simulink model "uz_ParameterID"  (R2021a)
settings: Solver=FixedStepDiscrete  StartTime=0.0  StopTime=160  FixedStep=0.000005  RelTol=1e-3  EnableMultiTasking=on
model workspace (MATLAB code in the model file):
  | cmdLim = Simulink.Parameter;
  | cmdLim.Value = 15;
  | cmdLim.Description = 'Limit for controlling the maximum surface command angle.';
  | cmdLim.Min = 0;
  | cmdLim.Max = 90;
  | cmdLim.DocUnits = 'deg';
  | 
  | dispGain = Simulink.Parameter;
  | dispGain.Value = 0.75;
  | dispGain.Description = 'Gain applied to the displacement error.';
  | dispGain.Min = 0;
  | dispGain.Max = [];
  | dispGain.DocUnits = 'deg/sec/deg';
  | 
  | dispLim = Simulink.Parameter;
  | dispLim.Value = 30;
  | dispLim.Description = 'Limit for controlling the maximum commanded angle.';
  | dispLim.Min = 0;
  | dispLim.Max = 180;
  | dispLim.DocUnits = 'deg';
  | 
  | intGain = Simulink.Parameter;
  | intGain.Value = 0.5;
  | intGain.Description = 'Gain applied to the integral error.';
  | intGain.Min = 0;
  | intGain.Max = [];
  | intGain.DocUnits = 'deg/sec/deg/sec';
  | 
  | intLim = Simulink.Parameter;
  | intLim.Value = 5;
  | intLim.Description = 'Limit for controlling the maximum commanded angle.';
  | intLim.Min = 0;
  | intLim.Max = 90;
  | intLim.DocUnits = 'deg';
  | 
  | rateGain = Simulink.Parameter;
  | rateGain.Value = 2;
  | rateGain.Description = 'Gain applied to the rate error.';
  | rateGain.Min = 0;
  | rateGain.Max = [];
  | rateGain.DocUnits = 'deg/deg/sec';
  | 
  | rateLim = Simulink.Parameter;
  | rateLim.Value = 6;
  | rateLim.Description = 'Limit for controlling the maximum commanded angle.';
  | rateLim.Min = 0;
  | rateLim.Max = 180;
  | rateLim.DocUnits = 'deg/sec';
  | 
  | hdgGain = Simulink.Parameter;
  | hdgGain.Value = 0.015;
values from neighbouring files (symbols this model uses):
  d_d_TMS = 0.005    [Parameter_Init_Buehler_201.m]
  d_f_hardware = 200000    [Parameter_Init_Buehler_201.m]
  d_f_states = 20000    [Parameter_Init_Buehler_201.m]
  d_i_max = 15    [Parameter_Init_Buehler_201.m]
  d_i_min = -d_i_max    (= -15)    [Parameter_Init_Buehler_201.m]
  d_I_n = 8    [Parameter_Init_Buehler_201.m]
  d_J_Coupling_M_E = 2e-6    (= 2e-06)    [Parameter_Init_Buehler_201.m]
  d_J_Coupling_M_Ms = 2e-20    [Parameter_Init_Buehler_201.m]
  d_J_Ms_L = d_J_Ms_M    (= 1.26363648e-05)    [Parameter_Init_Buehler_201.m]
  d_J_Ms_M = 0.5*0.5*((0.5*d_d_Ms)^4)*3.14*d_l_Ms*d_rho_Ms    (= 1.26363648e-05)    [Parameter_Init_Buehler_201.m]
  d_Ki_id = 162.47    [Parameter_Init_Buehler_201.m]
  d_Ki_iq = 162.47    [Parameter_Init_Buehler_201.m]
  d_Ki_n = 1.982    [Parameter_Init_Buehler_201.m]
  d_Kp_id = 0.369    [Parameter_Init_Buehler_201.m]
  d_Kp_iq = 0.369    [Parameter_Init_Buehler_201.m]
  d_Kp_n = 0.198    [Parameter_Init_Buehler_201.m]
  d_L_d = 0.00031    [Parameter_Init_Buehler_201.m]
  d_L_q = 0.00033    [Parameter_Init_Buehler_201.m]
  d_n_n = 3200    [Parameter_Init_Buehler_201.m]
  d_p = 4    [Parameter_Init_Buehler_201.m]
  d_psi_pm = 0.0075    [Parameter_Init_Buehler_201.m]
  d_R_ph = d_R_ph_ph/2    (= 0.089)    [Parameter_Init_Buehler_201.m]
  d_y_max = 10    [Parameter_Init_Buehler_201.m]
  d_y_min = -d_y_max    (= -10)    [Parameter_Init_Buehler_201.m]
undefined symbols (not defined in the file or in its folder): i_dq, i_dq_ref, n_ref, V_abc, v_dq
libraries: fl_lib x47, nesl_utility x30, ee_lib x18, simulink x8, spsabctodq0Lib x2, spsdq0toabcLib x1, spsTriangleGeneratorLib x1
(part 1 of 4)
settings Model: RequirementInfo={} %GIDa_fe9045fd_0412_4b6e_8206_617cc20e6fde  FPTRunName=Active  Creator=ts  LastModifiedBy=valen
settings SolverCC: AlgebraicLoopSolver=TrustRegion  PositivePriorityOrder=on  AutoInsertRateTranBlk=on
settings DataIOCC: SaveOutput=off  SignalLogging=off  DSMLogging=off  SaveTime=off
settings OptimizationCC: DefaultParameterBehavior=Inlined  UseDivisionForNetSlopeComputation=on  GainParamInheritBuiltInType=on  UseFloatMulNetSlope=on  DefaultUnderspecifiedDataType=single  UseSpecifiedMinMax=on  InlineInvariantSignals=on  PassReuseOutputArgsAs=Individual arguments  ZeroExternalMemoryAtStartup=off  ZeroInternalMemoryAtStartup=off  NoFixptDivByZeroProtection=on  EfficientFloat2IntCast=on  LifeSpan=1  MaxStackSize=64  OptimizeBlockOrder=speed  DifferentSizesBufferReuse=on  EfficientTunableParamExpr=on
settings DebuggingCC: BusObjectLabelMismatch=error  AllowSymbolicDim=off  SFUnexpectedBacktrackingDiag=warning  SFNoUnconditionalDefaultTransitionDiag=warning  SFExecutionAtInitializationDiag=none  SFMachineParentedDataDiag=warning  ArithmeticOperatorsInVariantConditions=warning
settings HardwareCC: ProdBitPerPointer=32  ProdBitPerSizeT=32  ProdBitPerPtrDiffT=32  ProdLargestAtomicInteger=Long  ProdLargestAtomicFloat=Double  ProdWordSize=32  ProdLongLongMode=on  ProdHWDeviceType=ARM Compatible->ARM Cortex-R  HardwareBoardFeatureSet=SoCBlockset
settings SFSimCC: SimGenImportedTypeDefs=on  MATLABDynamicMemAlloc=off
settings RTWCC: SystemTargetFile=ert.tlc  GenCodeOnly=on  TemplateMakefile=ert_default_tmf  GenerateReport=on  BuildConfiguration=Faster Runs  IncludeHyperlinkInReport=on  LaunchReport=on  GenerateTraceInfo=on  GenerateTraceReport=on  GenerateTraceReportSl=on  GenerateTraceReportSf=on  GenerateTraceReportEml=on  GenerateCodeMetricsReport=on  CheckMdlBeforeBuild=Warning
settings CodeAppCC: ForceParamTrailComments=on  IgnoreCustomStorageClasses=off  OperatorAnnotations=on  SimulinkDataObjDesc=on  SFDataObjDesc=on  MATLABFcnDesc=on  CustomSymbolStrGlobalVar=rt$M$R$N  CustomSymbolStrType=$N$M$R_t  CustomSymbolStrFcn=$N$M$F  CustomSymbolStrMacro=$N$M  InsertBlockDesc=on  StateflowObjectComments=on  MATLABSourceComments=on  EnableCustomComments=on  ReqsInCode=on
settings ERTTargetCC: TargetLangStandard=C99 (ISO)  CodeReplacementLibrary=GNU C99 extensions  MultiwordLength=2048  IncludeMdlTerminateFcn=off  CombineSignalStateStructs=on  SuppressErrorStatus=on  IncludeFileDelimiter=UseQuote  SupportAbsoluteTime=off  CodeInterfacePackaging=Reusable function  SupportNonFinite=off  RemoveResetFunc=off  InlinedParameterPlacement=NonHierarchical  MultiInstanceErrorCode=Warning  RootIOFormat=Part of model data structure  ERTCustomFileTemplate=example_file_process.tlc  GlobalDataDefinition=InSourceFile  GlobalDataReference=InSourceFile  ERTFilePackagingFormat=CompactWithDataFile  SuppressUnreachableDefaultCases=off
settings ConfigComp: CovScope=ReferencedModels  CovSaveName=covdata_rollAP  CovMetricSettings=dcmtrwe  CovHTMLOptions=-sRT=1 -aTS=1 -bRG=1 -bTC=1 -hTR=1 -nFC=0 -scm=1 -bcm=1 -xEv=0  CovSaveCumulativeToWorkspaceVar=on  CovSaveSingleToWorkspaceVar=on  CovCumulativeVarName=covCumulativeData_rollAP  CovReportOnPause=off  CovExternalEMLEnable=off  CovSFcnEnable=off

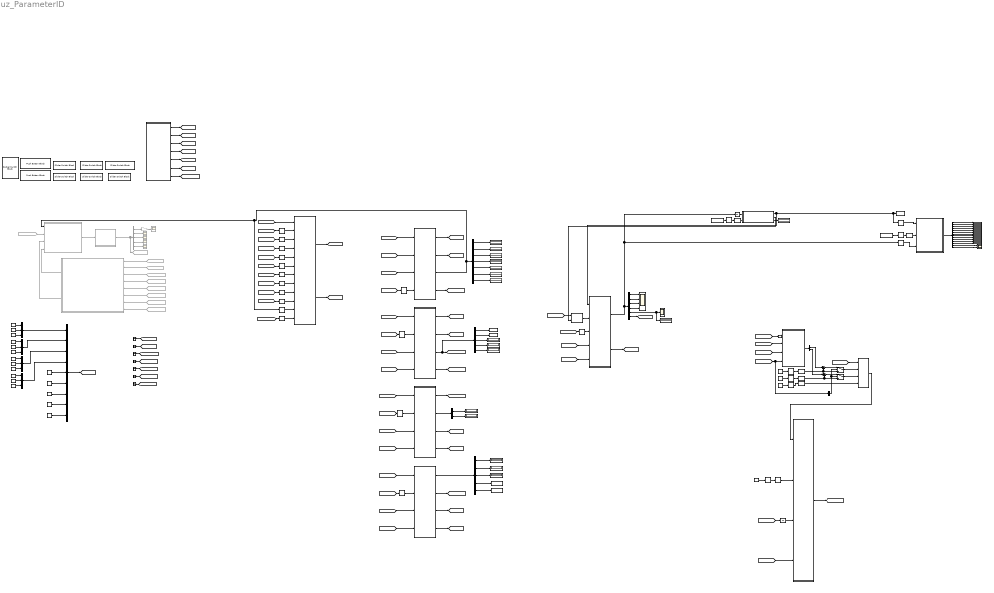
== system uz_ParameterID ==
  note: Description of Interpoaltion_Mesh_Grid:
      |
      | This function is calculating the regular flux maps out of the irregular scatter data array stored in psi_array_in. The outputs rangeX are containg the flux maps axis information, whereby the range is related to 3 times "i_rat" input.
      | Furthermore, the temperature dependency of the permanent flux is calculated if there are enough measuring values stored in the "delta_psi" array. The temperature constant as well as the estimated error of permanent flux,
      | at reference temperature, are given out on "psi_temp_const" and "psi_temp_error" outputs. Using this temperature dependency, the flux maps are updated with the permanent flux offset caused by the temperature which is given
      | in on "Wtemp_in" input.
  note: Stateflow for OnlineID
  note: part of main
  note: part of interupt service routine
  note: Software
  note: Hardware & FOC
  note: Description of clean_psi_array:
      |
      | This function is cleaning the array storing the measurement values, which always consits of a d-q-current combination a winding temperature and a speed value such as a d-q-flux combination
      | The function is searching for measuring pairs which are closer than "eta_c" to their neighbours. In this case it is averaging this similar pairs to avoid measuring values containing the same information.
      | This is essential for calculating a wide ranging flux map out of this array. Furthermore, there is an output "n_flux_points" giving back the amount of independent measuring pairs. This is the number (x/100) i show in the JavaGUI on the rigth top corner.
  note: Uncomment for code gen & Comment out hardware
  note: Description of ControlState:
      |
      | This state includes controls all the other states. It decides, based on user input, which state is executed and in which order. This is done via ControlFlags and finished/entered Flags of the individual states. If multiple ID's are requested, this state will automatically start the next one after the previous one has finished. This is an integral part of the ParameterID and must always be implemented.
  note: Description FOC_ControlState:
      |
      | This Stateflow is entered, after every other ID-state is finished (except OnlineID). It's just a simple state for current & speed control, depending on what the user chose in the config. This is only used to control the FOC with inputs after the ID-states are done. This state is solely used for simulation purposes.
  note: supporting states (can be, but don't have to be used. Mostly used for simulation)
  0 = current control 1 = speed control : Constant  Value=0
  AutoRefCurrents : Stateflow chart  TreatAsAtomicUnit=on
      settings: PortSchema="{\"entries\":[{\"content\":{\"sides\":[{\"content\":{\"connectorIds\":[\"In1\",\"In2\",\"In4\",\"In3\"]},\"type\":\"ConnectorPlacement.EquallySpacedRectSide\",\"uuid\":\"72ec0a24-315d-4dd0-9768-288ce3b452e0\"},{\"content\":{\"connectorIds\":[\"Out1\"],\"side\":\"RIGHT\"},\"type\":\"ConnectorPlacement.EquallySpacedRectSide\",\"uuid\":\"ab2b6233-d9cb-4afd-91e6-1fd664e04fd4\"},{\"content\":{\"connectorIds\":[],\"side\":\"TOP\"},\"type\":\"ConnectorPlacement.EquallySpacedRectSide\",\"uuid\":\"64b2df27-0928-499d-b44c-d4351b3511f9\"}]},\"type\":\"ConnectorPlacement.EquallySpacedConnector\",\"uuid\":\"4bb55e1f-14f7-4ef2-bb52-ee940a9b3e5d\"}],\"packageUris\":[\"http://schema.mathworks.com/mf0/Connector/R2020b\"],\"version\":\"1.0\"}"
  Bus Assignment : BusAssignment  AssignedSignals=i_dq_ref.d,i_dq_ref.q,n_ref
  Bus Assignment1 : BusAssignment  AssignedSignals=array_cleaned
  Bus Creator : BusCreator  Inputs=9  OutDataTypeStr=Bus: uz_ParaID_ActualValues_t
  Bus Creator1 : BusCreator  Inputs=3  OutDataTypeStr=Bus: uz_3ph_abc_t
  Bus Creator2 : BusCreator  Inputs=3  OutDataTypeStr=Bus: uz_3ph_abc_t
  Bus Creator3 : BusCreator  Inputs=3  OutDataTypeStr=Bus: uz_3ph_dq_t
  Bus Creator4 : BusCreator  Inputs=3  OutDataTypeStr=Bus: uz_3ph_dq_t
  Bus Selector : BusSelector  OutputSignals=BrkTorque,CoulTorque,ViscoTorque,measArrayTorque,measArraySpeed
  Bus Selector1 : BusSelector  Commented=on  OutputSignals=omega_m,i_dq,v_dq,I_abc,V_abc
  Bus Selector2 : BusSelector  OutputSignals=thetaOffset,PMSM_parameters.R_ph_Ohm,PMSM_parameters.Ld_Henry,PMSM_parameters.Lq_Henry,PMSM_parameters.Psi_PM_Vs,PMSM_parameters.J_kg_m_squared,PMSM_parameters.polePairs
  Bus Selector3 : BusSelector  OutputSignals=range_psid_X,range_psiq_X,range_id_X,range_iq_X,range_psid_Y,range_psiq_Y,range_id_Y,range_iq_Y,psiq_grid,psid_grid,id_grid,iq_grid,psi_temp_const,psi_temp_error
  Bus Selector4 : BusSelector  OutputSignals=i_dq_ref.d,i_dq_ref.q
  Bus Selector5 : BusSelector  OutputSignals=R_s,WindingTemp
  Bus Selector6 : BusSelector  OutputSignals=c_est_out,d_est_out,LoadInertia,TrainInertia,rotorInertia
  Bus Selector7 : BusSelector  OutputSignals=enableCRS
  Bus Selector8 : BusSelector  OutputSignals=Rph_out,Ld_out,Lq_out,psi_pm_out,activeState,id_out
  CleanPsiArray : MATLAB Function
  Const27 : Constant  Value=0.01*d_I_n
  Const53 : Constant  Value=d_I_n
  Const7 : Constant  Value=0.6
  Const8 : Constant  Value=0
  Const9 : Constant  Value=1000
  ControlState : Stateflow chart  TreatAsAtomicUnit=on
      settings: PortSchema="{\"entries\":[{\"content\":{\"sides\":[{\"content\":{\"connectorIds\":[\"In11\",\"In1\",\"In2\",\"In3\",\"In4\",\"In5\",\"In8\",\"In7\",\"In6\",\"In12\",\"In9\",\"In10\"]},\"type\":\"ConnectorPlacement.EquallySpacedRectSide\",\"uuid\":\"3338e9a8-28b4-45bb-be16-581ebbf0e7d5\"},{\"content\":{\"connectorIds\":[\"Out1\",\"Out2\"],\"side\":\"RIGHT\"},\"type\":\"ConnectorPlacement.EquallySpacedRectSide\",\"uuid\":\"68ffdf0a-d88e-422d-a36e-256c991e1a1a\"},{\"content\":{\"connectorIds\":[],\"side\":\"TOP\"},\"type\":\"ConnectorPlacement.EquallySpacedRectSide\",\"uuid\":\"571bf6fb-233c-470d-b735-d23e4cf83e69\"}]},\"type\":\"ConnectorPlacement.EquallySpacedConnector\",\"uuid\":\"829c5db0-50d3-4caf-9d4e-ee907b3905d4\"}],\"packageUris\":[\"http://schema.mathworks.com/mf0/Connector/R2020b\"],\"version\":\"1.0\"}"
  Data Type Conversion107 : DataTypeConversion  OutDataTypeStr=boolean
  Data Type Conversion{12..13,15,60,86} (5 alike) : DataTypeConversion  OutDataTypeStr=single
  Delay{,1..9,14} (11 alike) : Delay  DelayLength=1  InitialCondition=0
  Display{1..3,5..11} (10 alike) : Display
  FOC : Subsystem  Commented=on
  FOC_ControlState : Stateflow chart  TreatAsAtomicUnit=on
      settings: PortSchema="{\"entries\":[{\"content\":{\"sides\":[{\"content\":{\"connectorIds\":[\"In2\",\"In4\",\"In1\",\"In3\"]},\"type\":\"ConnectorPlacement.EquallySpacedRectSide\",\"uuid\":\"51616e24-a97c-4867-a832-fbf8995ba5af\"},{\"content\":{\"connectorIds\":[\"Out1\"],\"side\":\"RIGHT\"},\"type\":\"ConnectorPlacement.EquallySpacedRectSide\",\"uuid\":\"f89ef2d6-1fe7-4143-9573-492fc01180c7\"},{\"content\":{\"connectorIds\":[],\"side\":\"TOP\"},\"type\":\"ConnectorPlacement.EquallySpacedRectSide\",\"uuid\":\"2a1663ee-9e4b-4188-8f87-b811d0bf4173\"}]},\"type\":\"ConnectorPlacement.EquallySpacedConnector\",\"uuid\":\"7415555a-a8a9-4dd7-91ae-86382220971a\"}],\"packageUris\":[\"http://schema.mathworks.com/mf0/Connector/R2020b\"],\"version\":\"1.0\"}"
  From14 : From  Commented=on  GotoTag=ActualValues
  From20 : From  Commented=on  GotoTag=TwoMassID_FOC_output
  From21 : From  Commented=on  GotoTag=FrictionID_FOC_output
  From22 : From  Commented=on  GotoTag=ElectricalID_FOC_output
  From24 : From  Commented=on  GotoTag=FluxMapID_FOC_output
  From25 : From  Commented=on  GotoTag=FOCControl_output
  From4 : From  Commented=on  GotoTag=ControlFlags
  From41 : From  Commented=on  GotoTag=ElectricalID_FOC_output
  From53 : From  Commented=on  GotoTag=TwoMassID_output
  Gain : Gain  Commented=on  Gain=60/(2*pi)
  Goto3 : Goto  Commented=on  GotoTag=ActualValues
  Hardware : Subsystem  Commented=on
  I_U : Constant  Value=0  OutDataTypeStr=single
  I_V : Constant  Value=0  OutDataTypeStr=single
  I_W : Constant  Value=0  OutDataTypeStr=single
  I_abc : Scope  Commented=on
  InterpMeshGrid : MATLAB Function  TreatAsAtomicUnit=on
  OnlineActiveState : Scope
  Push Button2 : PushButtonBlock  ButtonText=RESET
  Push Button3 : PushButtonBlock  ButtonText=ACCEPT
  RT : RateTransition  OutPortSampleTime=0.0001
  Rate Transition : RateTransition  OutPortSampleTime=0.1
  Rate Transition{1..6,13..14,78,147} (10 alike) : RateTransition  OutPortSampleTime=1/d_f_states
  Rate Transition85 : RateTransition  OutPortSampleTime=0.1
  Rate Transition90 : RateTransition  OutPortSampleTime=0.1
  Rs,Ld,Lq,Psi_pm : Scope  NumInputPorts=4
  Scope2 : Scope  NumInputPorts=2
  Select Control : SliderSwitchBlock  LabelPosition=Hide
      settings: Values={{'Current', 'Speed'}, [0 1]}
  Subsystem Reference : Subsystem  ReferencedSubsystem=FrictionID
  Subsystem Reference1 : Subsystem  ReferencedSubsystem=FluxMapID
  Subsystem Reference2 : Subsystem  ReferencedSubsystem=ElectricalID
  Subsystem Reference3 : Subsystem  ReferencedSubsystem=TwoMassID
  Subsystem Reference4 : Subsystem  ReferencedSubsystem=OnlineID
  Sum : Sum  Inputs=|++
  Sum1 : Sum  Inputs=|++
  Switch2 : Switch  Criteria=u2 > Threshold
  Switch3 : Switch  Criteria=u2 > Threshold
  Terminator{,1..6} (7 alike) : Terminator
  To Workspace1 : ToWorkspace  VariableName=measArrayTorque  SampleTime=-1
      settings: MaxDataPoints=1
  To Workspace15 : ToWorkspace  VariableName=psi_array  SampleTime=-1
      settings: MaxDataPoints=1
  To Workspace16 : ToWorkspace  VariableName=rangepdX  SampleTime=-1
      settings: MaxDataPoints=1
  To Workspace17 : ToWorkspace  VariableName=rangepqX  SampleTime=-1
      settings: MaxDataPoints=1
  To Workspace18 : ToWorkspace  VariableName=rangeidX  SampleTime=-1
      settings: MaxDataPoints=1
  To Workspace19 : ToWorkspace  VariableName=rangeiqX  SampleTime=-1
      settings: MaxDataPoints=1
  To Workspace2 : ToWorkspace  VariableName=measArraySpeed  SampleTime=-1
      settings: MaxDataPoints=1
  To Workspace20 : ToWorkspace  VariableName=rangepdY  SampleTime=-1
      settings: MaxDataPoints=1
  To Workspace21 : ToWorkspace  VariableName=rangepqY  SampleTime=-1
      settings: MaxDataPoints=1
  To Workspace22 : ToWorkspace  VariableName=rangeidY  SampleTime=-1
      settings: MaxDataPoints=1
  To Workspace23 : ToWorkspace  VariableName=rangeiqY  SampleTime=-1
      settings: MaxDataPoints=1
  To Workspace24 : ToWorkspace  VariableName=psiq_grid  SampleTime=-1
      settings: MaxDataPoints=1
  To Workspace25 : ToWorkspace  VariableName=psid_grid  SampleTime=-1
      settings: MaxDataPoints=1
  To Workspace26 : ToWorkspace  VariableName=id_grid  SampleTime=-1
      settings: MaxDataPoints=1
  To Workspace27 : ToWorkspace  VariableName=iq_grid  SampleTime=-1
      settings: MaxDataPoints=1
  To Workspace31 : ToWorkspace  VariableName=c_est_out  SampleTime=-1
      settings: MaxDataPoints=1
  To Workspace32 : ToWorkspace  VariableName=d_est_out  SampleTime=-1
      settings: MaxDataPoints=1
  Unit Delay : UnitDelay  SampleTime=-1  HasFrameUpgradeWarning=on
  Unit Delay3 : UnitDelay  SampleTime=-1  HasFrameUpgradeWarning=on
  V_DC : Constant  Value=0  OutDataTypeStr=single
  V_U : Constant  Value=0  OutDataTypeStr=single
  V_V : Constant  Value=0  OutDataTypeStr=single
  V_W : Constant  Value=0  OutDataTypeStr=single
  V_abc : Scope  Commented=on
  config : Subsystem
  d-axis inductance Ld [H] : Display
  dqTrans : Subsystem  Commented=on
  enable ElectricalID : SliderSwitchBlock  LabelPosition=Hide
      settings: Values={{'Off', 'On'}, [0 1]}
  enable FluxMapID : SliderSwitchBlock  LabelPosition=Hide
      settings: Values={{'Off', 'On'}, [0 1]}
  enable FrictionID : SliderSwitchBlock  LabelPosition=Hide
      settings: Values={{'Off', 'On'}, [0 1]}
  enable OnlineID : SliderSwitchBlock  LabelPosition=Hide
      settings: Values={{'Off', 'On'}, [0 1]}
  enable TwoMassID : SliderSwitchBlock  LabelPosition=Hide
      settings: Values={{'Off', 'On'}, [0 1]}
  enableParameterID : RockerSwitchBlock  LabelPosition=Hide
      settings: Values={{'Off', 'On'}, [0 1]}
  i_d : Constant  Value=0  OutDataTypeStr=single
  i_d i_q : Scope  Commented=on
  i_q : Constant  Value=0  OutDataTypeStr=single
  i_zero : Constant  Value=0  OutDataTypeStr=single
  omega_el : Constant  Value=0  OutDataTypeStr=single
  omega_m : Constant  Value=0  OutDataTypeStr=single
  p : Display
  phase resistance [Ohm] : Display
  psiPM [Vs] : Display
  q-axis inductance Lq [H] : Display
  rotor speed [rpm] : Scope  Commented=on
  rotorInertia  [kg*m²] : Display
  thetaOffset [rad] : Display
  theta_el : Constant  Value=0  OutDataTypeStr=single
  theta_m : Constant  Value=0  OutDataTypeStr=single
  v_d : Constant  Value=0  OutDataTypeStr=single
  v_d v_q : Scope  Commented=on
  v_q : Constant  Value=0  OutDataTypeStr=single
  v_zero : Constant  Value=0  OutDataTypeStr=single
  wires:
  Bus Selector/3 -> Display10/1  "<ViscoTorque>"
  Sum/1 -> Switch3/1
  Const8/1 -> Rate Transition13/1
  config/5(TwoMassIDConfig) -> [TwoMassIDConfig]
  Bus Selector2/4 -> q-axis inductance Lq [H]/1  "<Lq_Henry>"
  [GlobalConfig] -> AutoRefCurrents/2(GlobalConfig)
  [finishedFrictionID] -> Delay/1
  Delay/1 -> ControlState/1(finishedFrictionID)
  Bus Selector2/5 -> psiPM [Vs]/1  "<Psi_PM_Vs>"
  Gain/1 -> rotor speed [rpm]/1
  Bus Selector8/1 -> Rs,Ld,Lq,Psi_pm/1  "<Rph_out>"
  Bus Selector6/5 -> Display6/1  "<rotorInertia>"
  Sum1/1 -> Switch2/1
  Const9/1 -> Rate Transition1/1
  Rate Transition14/1 -> Data Type Conversion13/1
  config/1(GlobalConfig) -> [GlobalConfig_in]
  Delay14/1 -> ControlState/9(ElectricalID_output)
  Delay2/1 -> ControlState/6(enteredFluxMapID)
  From24/1 -> FOC/5(FluxMapID_FOC_input)
  Delay5/1 -> ControlState/8(enteredElectricalID)
  Delay6/1 -> ControlState/7(enteredTwoMassID)
  [enteredElectricalID] -> Delay5/1
  Rate Transition85/1 -> Data Type Conversion86/1
  [enteredFrictionID] -> Delay1/1
  From25/1 -> FOC/6(FOCControl_input)
  Data Type Conversion13/1 -> Sum1/2, Switch2/3  "i_q_ref"
  Rate Transition90/1 -> InterpMeshGrid/3(OnlineID_input)
  [finishedFluxMapID] -> Delay4/1
  [finishedTwoMassID] -> Delay3/1
  FOC/2(PWM_out) -> Hardware/3(PWM_FOC_in)
  [ActualValues] -> RT/1
  Bus Selector1/1 -> Gain/1  "<omega_m>"
  config/2(ElectricalIDConfig) -> [ElectricalIDConfig]
  config/4(FrictionIDConfig) -> [FrictionIDConfig]
  Const53/1 -> Rate Transition85/1
  Const27/1 -> Rate Transition78/1
  Data Type Conversion60/1 -> CleanPsiArray/2(eta_c)
  Bus Selector2/6 -> rotorInertia  [kg*m²]/1  "<J_kg_m_squared>"
  Bus Selector/1 -> Display11/1  "<BrkTorque>"
  Delay1/1 -> ControlState/5(enteredFrictionID)
  Bus Selector2/7 -> p/1  "<polePairs>"
  [ElectricalID_FOC_output] -> Delay8/1
  Rate Transition13/1 -> Data Type Conversion12/1
  Unit Delay/1 -> FOC_ControlState/1(i_d_Online_ref)
  Rate Transition/1 -> InterpMeshGrid/1(psi_array_in)
  Delay7/1 -> ControlState/2(finishedElectricalID)
  Bus Selector2/2 -> phase resistance [Ohm]/1  "<R_ph_Ohm>"
  Bus Selector2/3 -> d-axis inductance Ld [H]/1  "<Ld_Henry>"
  [ActualValues] -> Rate Transition6/1
  Delay8/1 -> ControlState/10(ElectricalID_FOC_output)
  Bus Selector6/3 -> Display3/1  "<LoadInertia>"
  ControlState/1(GlobalConfig_out) -> [GlobalConfig]
  From4/1 -> FOC/1(ControlFlags)
  [ActualValues] -> Rate Transition2/1
  config/6(OnlineIDConfig) -> [OnlineIDConfig]
  [ActualValues] -> Rate Transition3/1
  CleanPsiArray/2(array_cleaned_flag) -> Bus Assignment1/2
  Bus Selector5/1 -> Display1/1  "<R_s>"
  [GlobalConfig_in] -> ControlState/11(GlobalConfig_in)
  [ControlFlags] -> FOC_ControlState/3(ControlFlags)
  From41/1 -> Hardware/2(ElectricalID_FOC_output)
  Const7/1 -> Rate Transition14/1
  Bus Selector6/4 -> Display5/1  "<TrainInertia>"
  Hardware/1(ActualValues) -> dqTrans/1(ActualValues)
  Data Type Conversion86/1 -> InterpMeshGrid/2(i_rat)
  Bus Selector8/4 -> Rs,Ld,Lq,Psi_pm/4  "<psi_pm_out>"
  Bus Selector8/2 -> Rs,Ld,Lq,Psi_pm/2  "<Ld_out>"
  Unit Delay3/1 -> CleanPsiArray/1(OnlineID_output)
  [OnlineIDConfig] -> Bus Assignment1/1
  From20/1 -> FOC/7(TwoMassID_FOC_input)
  Rate Transition78/1 -> Data Type Conversion60/1
  Rate Transition1/1 -> Data Type Conversion15/1
  Bus Selector8/5 -> Display8/1, OnlineActiveState/1  "<activeState>"
  Delay3/1 -> ControlState/3(finishedTwoMassID)
  CleanPsiArray/1(psi_array_out) -> Subsystem Reference4/1, Rate Transition/1, To Workspace15/1  "cleaned_psi_array"
  FOC/1(FOC_enable_out) -> Hardware/4(FOC_enabled)
  Bus Selector2/1 -> thetaOffset [rad]/1  "<thetaOffset>"
  config/3(FluxMapIDConfig) -> [FluxMapIDConfig]
  From21/1 -> FOC/3(FrictionID_FOC_input)
  Bus Selector1/2 -> i_d i_q/1  "<i_dq>"
  CleanPsiArray/3(n_flux_points) -> Display7/1
  Bus Selector/2 -> Display9/1  "<CoulTorque>"
  ControlState/2(ControlFlags) -> [ControlFlags]
  [ActualValues] -> Rate Transition4/1
  Bus Selector6/1 -> To Workspace31/1  "<c_est_out>"
  Bus Selector6/2 -> To Workspace32/1  "<d_est_out>"
  FOC_ControlState/1(FOCControl_output) -> [FOCControl_output]
  Delay4/1 -> ControlState/4(finishedFluxMapID)
  [finishedElectricalID] -> Delay7/1
  From22/1 -> FOC/4(ElectricalID_FOC_input)
  Bus Assignment/1 -> FOC_ControlState/2(GlobalConfig)
  [ActualValues] -> Rate Transition5/1
  Bus Selector8/3 -> Rs,Ld,Lq,Psi_pm/3  "<Lq_out>"
  Data Type Conversion12/1 -> Switch3/3, Sum/2  "i_d_ref"
  [enteredFluxMapID] -> Delay2/1
  From14/1 -> FOC/2(ActualValues)
  [enteredTwoMassID] -> Delay6/1
  Bus Selector5/2 -> Display2/1  "<WindingTemp>"
  [ActualValues] -> Terminator/1
  [TwoMassID_FOC_output] -> Terminator6/1
  [FrictionID_FOC_output] -> Terminator2/1
  [ElectricalID_FOC_output] -> Terminator3/1
  [FluxMapID_FOC_output] -> Terminator4/1
  [ControlFlags] -> Terminator1/1
  [FOCControl_output] -> Terminator5/1
  omega_el/1 -> Bus Creator/6  "omega_el"
  Bus Creator/1 -> [ActualValues]
  omega_m/1 -> Bus Creator/5  "omega_m"
  theta_m/1 -> Bus Creator/7  "theta_m"
  V_DC/1 -> Bus Creator/9  "V_DC"
  V_V/1 -> Bus Creator1/2  "b"
  V_U/1 -> Bus Creator1/1  "a"
  V_W/1 -> Bus Creator1/3  "c"
  Bus Creator1/1 -> Bus Creator/1  "V_abc"
  Bus Creator2/1 -> Bus Creator/2  "I_abc"
  I_V/1 -> Bus Creator2/2  "b"
  I_U/1 -> Bus Creator2/1  "a"
  I_W/1 -> Bus Creator2/3  "c"
  Bus Creator3/1 -> Bus Creator/4  "v_dq"
  v_q/1 -> Bus Creator3/2  "q"
  v_d/1 -> Bus Creator3/1  "d"
  v_zero/1 -> Bus Creator3/3  "zero"
  Bus Creator4/1 -> Bus Creator/3  "i_dq"
  i_q/1 -> Bus Creator4/2  "q"
  i_d/1 -> Bus Creator4/1  "d"
  i_zero/1 -> Bus Creator4/3  "zero"
  Bus Selector1/3 -> v_d v_q/1  "<v_dq>"
  Bus Selector1/4 -> I_abc/1  "<I_abc>"
  Bus Selector1/5 -> V_abc/1  "<V_abc>"
  theta_el/1 -> Bus Creator/8  "theta_el"
  [GlobalConfig] -> Bus Assignment/1
  Switch2/1 -> Bus Assignment/3
  Switch3/1 -> Bus Assignment/2
  Data Type Conversion15/1 -> Bus Assignment/4  "n_ref"
  RT/1 -> AutoRefCurrents/1(ActualValues)
  Bus Selector8/6 -> [OnlineID_id_out]  "<id_out>"
  [OnlineID_id_out] -> Unit Delay/1
  Rate Transition147/1 -> Data Type Conversion107/1
  Data Type Conversion107/1 -> FOC_ControlState/4(controlType)  "controlType"
  0 = current control 1 = speed control/1 -> Rate Transition147/1
  Bus Selector3/1 -> To Workspace16/1  "<range_psid_X>"
  Bus Selector3/2 -> To Workspace17/1  "<range_psiq_X>"
  InterpMeshGrid/1(FluxMapData) -> Bus Selector3/1
  Bus Selector3/14 -> Scope2/2  "<psi_temp_error>"
  Bus Selector3/13 -> Scope2/1  "<psi_temp_const>"
  Bus Selector3/3 -> To Workspace18/1  "<range_id_X>"
  Bus Selector3/4 -> To Workspace19/1  "<range_iq_X>"
  Bus Selector3/5 -> To Workspace20/1  "<range_psid_Y>"
  Bus Selector3/6 -> To Workspace21/1  "<range_psiq_Y>"
  Bus Selector3/7 -> To Workspace22/1  "<range_id_Y>"
  Bus Selector3/8 -> To Workspace23/1  "<range_iq_Y>"
  Bus Selector3/9 -> To Workspace24/1  "<psiq_grid>"
  Bus Selector3/10 -> To Workspace25/1  "<psid_grid>"
  Bus Selector3/11 -> To Workspace26/1  "<id_grid>"
  Bus Selector3/12 -> To Workspace27/1  "<iq_grid>"
  config/7(AutoRefCurrentsconfig) -> [AutoRefCurrentsConfig]
  [AutoRefCurrentsConfig] -> Bus Selector7/1, AutoRefCurrents/3(AutoRefCurrentsConfig)
  AutoRefCurrents/1(AutoRefCurrents_output) -> Bus Selector4/1
  Bus Selector4/1 -> Sum/1  "<d>"
  Bus Selector4/2 -> Sum1/1  "<q>"
  Bus Selector7/1 -> Switch2/2, Switch3/2  "<enableCRS>"
  [ControlFlags] -> AutoRefCurrents/4(ControlFlags)
  Delay9/1 -> ControlState/12(enteredOnlineID)
  [enteredOnlineID] -> Delay9/1
  From53/1 -> FOC/8(ElectricalID_FOC_input1)
  Bus Selector/4 -> To Workspace1/1  "<measArrayTorque>"
  Bus Selector/5 -> To Workspace2/1  "<measArraySpeed>"
  dqTrans/1(ActualValues_corr) -> Goto3/1, Bus Selector1/1
  [FrictionIDConfig] -> Subsystem Reference/1
  Rate Transition5/1 -> Subsystem Reference/2
  [GlobalConfig] -> Subsystem Reference/3
  [ControlFlags] -> Subsystem Reference/4
  Subsystem Reference/1 -> Bus Selector/1
  Subsystem Reference/2 -> [FrictionID_FOC_output]
  Subsystem Reference/3 -> [enteredFrictionID]
  Subsystem Reference/4 -> [finishedFrictionID]
  [FluxMapIDConfig] -> Subsystem Reference1/1
  Rate Transition4/1 -> Subsystem Reference1/2
  [GlobalConfig] -> Subsystem Reference1/3
  [ControlFlags] -> Subsystem Reference1/4
  Subsystem Reference1/1 -> [FluxMapID_FOC_output]
  Subsystem Reference1/2 -> Bus Selector5/1
  Subsystem Reference1/3 -> [finishedFluxMapID]
  Subsystem Reference1/4 -> [enteredFluxMapID]
  Subsystem Reference2/3 -> Hardware/1(ElectricalID_output), Delay14/1, Bus Selector2/1
  [GlobalConfig] -> Subsystem Reference2/1
  [ControlFlags] -> Subsystem Reference2/2
  [ElectricalIDConfig] -> Subsystem Reference2/3
  Rate Transition6/1 -> Subsystem Reference2/4
  Subsystem Reference2/1 -> [enteredElectricalID]
  Subsystem Reference2/2 -> [finishedElectricalID]
  Subsystem Reference2/4 -> [ElectricalID_FOC_output]
  Subsystem Reference3/3 -> Bus Selector6/1, [TwoMassID_output]
  [TwoMassIDConfig] -> Subsystem Reference3/1
  Rate Transition2/1 -> Subsystem Reference3/2
  [GlobalConfig] -> Subsystem Reference3/3
  [ControlFlags] -> Subsystem Reference3/4
  Subsystem Reference3/1 -> [finishedTwoMassID]
  Subsystem Reference3/2 -> [enteredTwoMassID]
  Subsystem Reference3/4 -> [TwoMassID_FOC_output]
  Subsystem Reference4/1 -> Unit Delay3/1, Rate Transition90/1, Bus Selector8/1
  Bus Assignment1/1 -> Subsystem Reference4/2
  Rate Transition3/1 -> Subsystem Reference4/3
  [GlobalConfig] -> Subsystem Reference4/4
  [ControlFlags] -> Subsystem Reference4/5
  Subsystem Reference4/2 -> [enteredOnlineID]

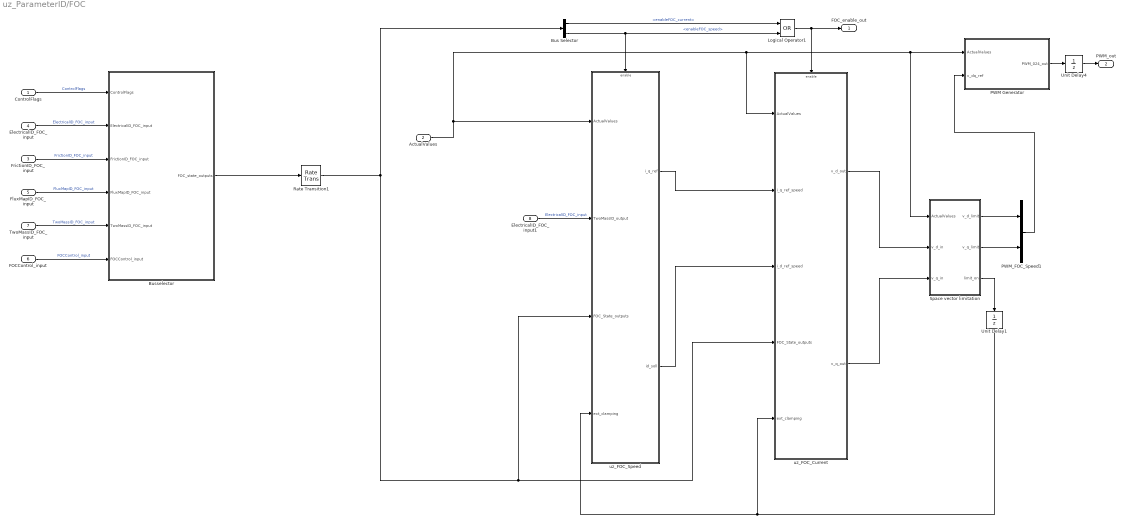
== system uz_ParameterID/FOC ==
  ControlFlags : Inport
  ActualValues : Inport  Port=2
  FrictionID_FOC_input : Inport  Port=3
  ElectricalID_FOC_input : Inport  Port=4
  FluxMapID_FOC_input : Inport  Port=5
  FOCControl_input : Inport  Port=6
  TwoMassID_FOC_input : Inport  Port=7
  ElectricalID_FOC_input1 : Inport  Port=8  OutDataTypeStr=Bus: uz_ParaID_TwoMassID_output_t
  Bus Selector : BusSelector  OutputSignals=enableFOC_current,enableFOC_speed
  Busselector : MATLAB Function  TreatAsAtomicUnit=on
  Logical Operator1 : Logic  Operator=OR  AllPortsSameDT=off  OutDataTypeStr=boolean
  PWM Generator : Subsystem
  PWM_FOC_Speed1 : Mux  Inputs=2
  Rate Transition1 : RateTransition  OutPortSampleTime=1/d_f_hardware
  Space vector limitation : MATLAB Function  TreatAsAtomicUnit=on
  Unit Delay1 : UnitDelay  SampleTime=-1  HasFrameUpgradeWarning=on
  Unit Delay4 : UnitDelay  SampleTime=-1  HasFrameUpgradeWarning=on
  uz_FOC_Current : Subsystem  SystemSampleTime=0.00001
  uz_FOC_Speed : Subsystem
  FOC_enable_out : Outport
  PWM_out : Outport  Port=2
  wires:
  FrictionID_FOC_input/1 -> Busselector/3(FrictionID_FOC_input)  "FrictionID_FOC_input"
  Bus Selector/1 -> Logical Operator1/1  "<enableFOC_current>"
  Bus Selector/2 -> Logical Operator1/2, uz_FOC_Speed/Enable  "<enableFOC_speed>"
  FOCControl_input/1 -> Busselector/6(FOCControl_input)  "FOCControl_input"
  ActualValues/1 -> Space vector limitation/1(ActualValues), PWM Generator/1(ActualValues), uz_FOC_Current/1(ActualValues), uz_FOC_Speed/1(ActualValues)
  TwoMassID_FOC_input/1 -> Busselector/5(TwoMassID_FOC_input)  "TwoMassID_FOC_input"
  FluxMapID_FOC_input/1 -> Busselector/4(FluxMapID_FOC_input)  "FluxMapID_FOC_input"
  Rate Transition1/1 -> Bus Selector/1, uz_FOC_Speed/3(FOC_State_outputs), uz_FOC_Current/4(FOC_State_outputs)
  ElectricalID_FOC_input/1 -> Busselector/2(ElectricalID_FOC_input)  "ElectricalID_FOC_input"
  ControlFlags/1 -> Busselector/1(ControlFlags)  "ControlFlags"
  PWM Generator/1(PWM_024_out) -> Unit Delay4/1
  Unit Delay4/1 -> PWM_out/1
  uz_FOC_Speed/1(i_q_ref) -> uz_FOC_Current/2(i_q_ref_speed)
  uz_FOC_Speed/2(id_soll) -> uz_FOC_Current/3(i_d_ref_speed)
  Logical Operator1/1 -> uz_FOC_Current/Enable, FOC_enable_out/1
  uz_FOC_Current/1(v_d_out) -> Space vector limitation/2(v_d_in)
  uz_FOC_Current/2(v_q_out) -> Space vector limitation/3(v_q_in)
  Space vector limitation/2(v_q_limit) -> PWM_FOC_Speed1/2
  Space vector limitation/1(v_d_limit) -> PWM_FOC_Speed1/1
  Space vector limitation/3(limit_on) -> Unit Delay1/1
  Unit Delay1/1 -> uz_FOC_Speed/4(ext_clamping), uz_FOC_Current/5(ext_clamping)
  PWM_FOC_Speed1/1 -> PWM Generator/2(v_dq_ref)
  Busselector/1(FOC_state_outputs) -> Rate Transition1/1
  ElectricalID_FOC_input1/1 -> uz_FOC_Speed/2(TwoMassID_output)  "ElectricalID_FOC_input"
